simulink model "rectify"  (R2022a)
settings: Solver=VariableStepAuto  StartTime=0.0  StopTime=10.0  RelTol=1e-3
settings Model: Creator=Tsing  LastModifiedBy=Tsing

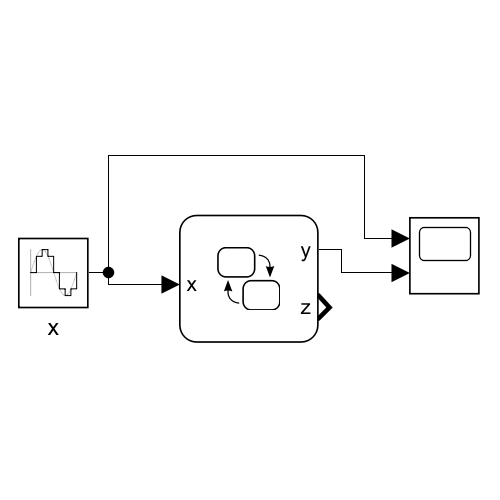
[thumbnail: Simulink's stored preview of the top-level diagram]
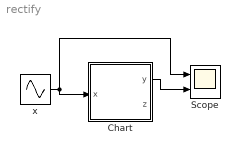
== system rectify ==
  Chart : Stateflow chart  TreatAsAtomicUnit=on
  Scope : Scope  NumInputPorts=2
  x : Sin  SampleTime=0.2
  wires:
  x/1 -> Scope/1, Chart/1(x)
  Chart/1(y) -> Scope/2

== stateflow chart rectify/Chart ==
  state On
    y = x;
    z = -x;
  state Off
    y = 0;
    z = 0;
  (default) -> On
  On -> Off : [x<t0]
  Off -> On : [x>=t0]
  data: x input; y output; t0 constant double =0; z output
